simulink model "Example_4_3"  (R2021b)
settings: Solver=VariableStepAuto  StartTime=0.0  StopTime=10  RelTol=1e-3
settings Model: Creator=saeed  LastModifiedBy=saeed

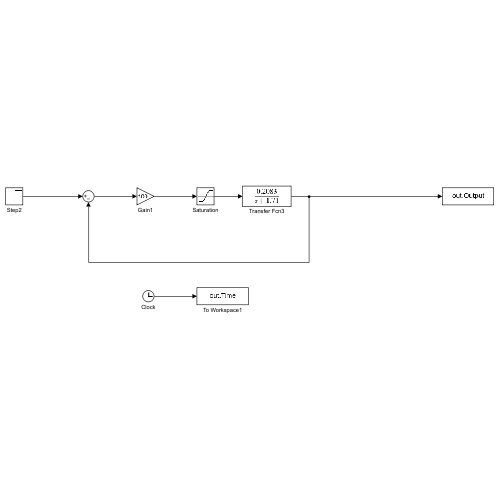
[thumbnail: Simulink's stored preview of the top-level diagram]
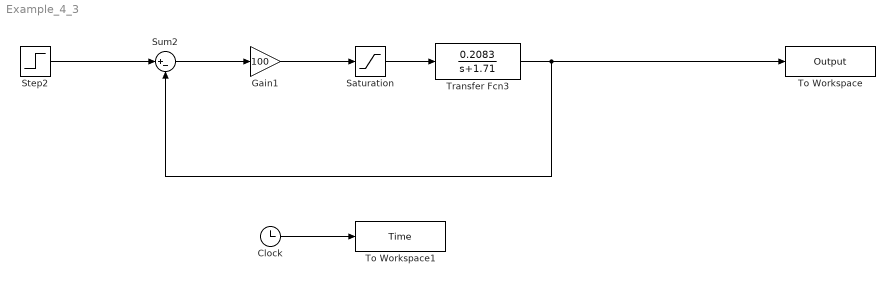
== system Example_4_3 ==
  Clock : Clock
  Gain1 : Gain  Gain=100
  Saturation : Saturate  UpperLimit=5  LowerLimit=-5
  Step2 : Step  Time=0  After=10  SampleTime=0
  Sum2 : Sum  Inputs=|+-
  To Workspace : ToWorkspace  VariableName=Output  SaveFormat=Timeseries  SampleTime=-1
  To Workspace1 : ToWorkspace  VariableName=Time  SaveFormat=Timeseries  SampleTime=-1
  Transfer Fcn3 : TransferFcn  Numerator=[0.2083]  Denominator=[1 1.71]
  wires:
  Step2/1 -> Sum2/1
  Sum2/1 -> Gain1/1
  Gain1/1 -> Saturation/1
  Saturation/1 -> Transfer Fcn3/1
  Transfer Fcn3/1 -> To Workspace/1, Sum2/2
  Clock/1 -> To Workspace1/1
